simulink model "cllc_control"  (R2022a)
settings: Solver=FixedStepDiscrete  StartTime=0.0  StopTime=Inf  FixedStep=stepsize  RelTol=1e-9  AbsTol=1e-9  EnableMultiTasking=on
model workspace (MAT data in the model file):
  A_d = [1 2 1 2 1 2 1 2 1 2 1 2 ... (18 elements, 2x9)]
  dcdc_direction = 1
  iout_ref : Simulink.Parameter (value not decoded)
  llc1_pri_idc : Simulink.Signal (value not decoded)
  llc1_sec_idc : Simulink.Signal (value not decoded)
  ref_iout : Simulink.Signal (value not decoded)
  ref_iout_calib : Simulink.Signal (value not decoded)
  ref_ss_llc1 : Simulink.Signal (value not decoded)
  ref_vbat : Simulink.Signal (value not decoded)
  ref_vbat_calib : Simulink.Signal (value not decoded)
  vbat : Simulink.Signal (value not decoded)
  vbat_ref : Simulink.Parameter (value not decoded)
  vout : Simulink.Signal (value not decoded)
values from neighbouring files (symbols this model uses):
  epwmclk = 100000000.0    [cllc_data_lib.sldd]
  stepsize = 2.0E-7    [cllc_data_lib.sldd]
  var_dir_v2g = 0.0    [cllc_data_lib.sldd]
undefined symbols (not defined in the file or in its folder): f32Iout, f32VoutTarget
libraries: spsSampleandHoldLib x16, simulink_extras x6
(part 2 of 2)

== system cllc_control/TI_F28379/epwm_cllc1/EPWM_AQCSFRC_SEC_QD ==
  maindrive : Inport
  epwm_aqcsfrc_csf : Inport  Port=2
  synci : Inport  Port=3
  Cast To Boolean : DataTypeConversion  OutDataTypeStr=boolean  SaturateOnIntegerOverflow=off  RndMeth=Floor
  NOT4 : Logic  Operator=NOT  IconShape=distinctive  AllPortsSameDT=off  OutDataTypeStr=boolean
  Product2 : Product
  Sample and Hold1 : spsSampleandHoldLib/Sample and Hold  ic=0  Ts=0
      settings: SourceProductBaseCode=PS
  maindrive' : Outport  PortDimensions=[1 1]
  wires:
  Cast To Boolean/1 -> maindrive'/1
  Sample and Hold1/1 -> Product2/2
  Product2/1 -> Cast To Boolean/1
  synci/1 -> Sample and Hold1/2
  NOT4/1 -> Sample and Hold1/1
  maindrive/1 -> Product2/1
  epwm_aqcsfrc_csf/1 -> NOT4/1

== system cllc_control/TI_F28379/epwm_cllc1/tb_updown ==
  Ts : Inport
  stepsize : Inport  Port=2
  Data Store Memory1 : DataStoreMemory  DataStoreName=sum  ReadBeforeWriteMsg=warning  WriteAfterWriteMsg=warning  WriteAfterReadMsg=warning  ShowAdditionalParam=off  OutDataTypeStr=double
  Data Store Read2 : DataStoreRead  DataStoreName=sum  IndexOptions=Index vector (dialog)  Indices=1  OutputSizes=1
  Data Store Write2 : DataStoreWrite  DataStoreName=sum  IndexOptions=Index vector (dialog)  Indices=1  OutputSizes=1
  MATLAB Function1 : MATLAB Function  Commented=on  TreatAsAtomicUnit=on
  MATLAB Function7 : MATLAB Function  TreatAsAtomicUnit=on
  tb_updown : Outport
  wires:
  Data Store Read2/1 -> MATLAB Function7/1(sum)
  MATLAB Function7/1(updown) -> Data Store Write2/1, tb_updown/1
  Ts/1 -> MATLAB Function7/2(Ts)
  stepsize/1 -> MATLAB Function7/3(stepsize)

== system cllc_control/TI_F28379/epwm_cllc1/tb_updown_ps ==
  Ts : Inport  OutDataTypeStr=double
  stepsize : Inport  Port=2  OutDataTypeStr=double
  synci : Inport  Port=3  OutDataTypeStr=double
  ps : Inport  Port=4  OutDataTypeStr=double
  Data Store Memory1 : DataStoreMemory  DataStoreName=sum2  ReadBeforeWriteMsg=warning  WriteAfterWriteMsg=warning  WriteAfterReadMsg=warning  ShowAdditionalParam=off  OutDataTypeStr=double
  Data Store Read2 : DataStoreRead  DataStoreName=sum2  IndexOptions=Index vector (dialog)  Indices=1  OutputSizes=1
  Data Store Write2 : DataStoreWrite  DataStoreName=sum2  IndexOptions=Index vector (dialog)  Indices=1  OutputSizes=1
  MATLAB Function7 : MATLAB Function  TreatAsAtomicUnit=on
  tb_updown : Outport  OutDataTypeStr=double
  wires:
  stepsize/1 -> MATLAB Function7/3(stepsize)
  Ts/1 -> MATLAB Function7/2(Ts)
  MATLAB Function7/1(updown) -> tb_updown/1, Data Store Write2/1
  Data Store Read2/1 -> MATLAB Function7/1(sum)
  synci/1 -> MATLAB Function7/4(synci)
  ps/1 -> MATLAB Function7/5(ps)

== system cllc_control/TI_F28379/epwm_cllc2/EPWM_AQCSFRC_PRI_QA ==
  maindrive : Inport
  epwm_aqcsfrc_csf : Inport  Port=2
  synci : Inport  Port=3
  Cast To Boolean : DataTypeConversion  OutDataTypeStr=boolean  SaturateOnIntegerOverflow=off  RndMeth=Floor
  NOT4 : Logic  Operator=NOT  IconShape=distinctive  AllPortsSameDT=off  OutDataTypeStr=boolean
  Product2 : Product
  Sample and Hold1 : spsSampleandHoldLib/Sample and Hold  ic=0  Ts=0
      settings: SourceProductBaseCode=PS
  maindrive' : Outport  PortDimensions=[1 1]
  wires:
  Cast To Boolean/1 -> maindrive'/1
  Sample and Hold1/1 -> Product2/2
  Product2/1 -> Cast To Boolean/1
  synci/1 -> Sample and Hold1/2
  NOT4/1 -> Sample and Hold1/1
  maindrive/1 -> Product2/1
  epwm_aqcsfrc_csf/1 -> NOT4/1

== system cllc_control/TI_F28379/epwm_cllc2/EPWM_AQCSFRC_PRI_QB ==
  maindrive : Inport
  epwm_aqcsfrc_csf : Inport  Port=2
  synci : Inport  Port=3
  Cast To Boolean : DataTypeConversion  OutDataTypeStr=boolean  SaturateOnIntegerOverflow=off  RndMeth=Floor
  NOT4 : Logic  Operator=NOT  IconShape=distinctive  AllPortsSameDT=off  OutDataTypeStr=boolean
  Product2 : Product
  Sample and Hold1 : spsSampleandHoldLib/Sample and Hold  ic=0  Ts=0
      settings: SourceProductBaseCode=PS
  maindrive' : Outport  PortDimensions=[1 1]
  wires:
  Cast To Boolean/1 -> maindrive'/1
  epwm_aqcsfrc_csf/1 -> NOT4/1
  maindrive/1 -> Product2/1
  NOT4/1 -> Sample and Hold1/1
  synci/1 -> Sample and Hold1/2
  Product2/1 -> Cast To Boolean/1
  Sample and Hold1/1 -> Product2/2

== system cllc_control/TI_F28379/epwm_cllc2/EPWM_AQCSFRC_PRI_QC ==
  maindrive : Inport
  epwm_aqcsfrc_csf : Inport  Port=2
  synci : Inport  Port=3
  Cast To Boolean : DataTypeConversion  OutDataTypeStr=boolean  SaturateOnIntegerOverflow=off  RndMeth=Floor
  NOT4 : Logic  Operator=NOT  IconShape=distinctive  AllPortsSameDT=off  OutDataTypeStr=boolean
  Product2 : Product
  Sample and Hold1 : spsSampleandHoldLib/Sample and Hold  ic=0  Ts=0
      settings: SourceProductBaseCode=PS
  maindrive' : Outport  PortDimensions=[1 1]
  wires:
  Cast To Boolean/1 -> maindrive'/1
  epwm_aqcsfrc_csf/1 -> NOT4/1
  maindrive/1 -> Product2/1
  NOT4/1 -> Sample and Hold1/1
  synci/1 -> Sample and Hold1/2
  Product2/1 -> Cast To Boolean/1
  Sample and Hold1/1 -> Product2/2

== system cllc_control/TI_F28379/epwm_cllc2/EPWM_AQCSFRC_PRI_QD ==
  maindrive : Inport
  epwm_aqcsfrc_csf : Inport  Port=2
  synci : Inport  Port=3
  Cast To Boolean : DataTypeConversion  OutDataTypeStr=boolean  SaturateOnIntegerOverflow=off  RndMeth=Floor
  NOT4 : Logic  Operator=NOT  IconShape=distinctive  AllPortsSameDT=off  OutDataTypeStr=boolean
  Product2 : Product
  Sample and Hold1 : spsSampleandHoldLib/Sample and Hold  ic=0  Ts=0
      settings: SourceProductBaseCode=PS
  maindrive' : Outport  PortDimensions=[1 1]
  wires:
  Cast To Boolean/1 -> maindrive'/1
  Sample and Hold1/1 -> Product2/2
  Product2/1 -> Cast To Boolean/1
  synci/1 -> Sample and Hold1/2
  NOT4/1 -> Sample and Hold1/1
  maindrive/1 -> Product2/1
  epwm_aqcsfrc_csf/1 -> NOT4/1

== system cllc_control/TI_F28379/epwm_cllc2/EPWM_AQCSFRC_SEC_QA ==
  maindrive : Inport
  epwm_aqcsfrc_csf : Inport  Port=2
  synci : Inport  Port=3
  Cast To Boolean : DataTypeConversion  OutDataTypeStr=boolean  SaturateOnIntegerOverflow=off  RndMeth=Floor
  NOT4 : Logic  Operator=NOT  IconShape=distinctive  AllPortsSameDT=off  OutDataTypeStr=boolean
  Product2 : Product
  Sample and Hold1 : spsSampleandHoldLib/Sample and Hold  ic=0  Ts=0
      settings: SourceProductBaseCode=PS
  maindrive' : Outport  PortDimensions=[1 1]
  wires:
  epwm_aqcsfrc_csf/1 -> NOT4/1
  maindrive/1 -> Product2/1
  NOT4/1 -> Sample and Hold1/1
  synci/1 -> Sample and Hold1/2
  Product2/1 -> Cast To Boolean/1
  Sample and Hold1/1 -> Product2/2
  Cast To Boolean/1 -> maindrive'/1

== system cllc_control/TI_F28379/epwm_cllc2/EPWM_AQCSFRC_SEC_QB ==
  maindrive : Inport
  epwm_aqcsfrc_csf : Inport  Port=2
  synci : Inport  Port=3
  Cast To Boolean : DataTypeConversion  OutDataTypeStr=boolean  SaturateOnIntegerOverflow=off  RndMeth=Floor
  NOT4 : Logic  Operator=NOT  IconShape=distinctive  AllPortsSameDT=off  OutDataTypeStr=boolean
  Product2 : Product
  Sample and Hold1 : spsSampleandHoldLib/Sample and Hold  ic=0  Ts=0
      settings: SourceProductBaseCode=PS
  maindrive' : Outport  PortDimensions=[1 1]
  wires:
  Sample and Hold1/1 -> Product2/2
  Product2/1 -> Cast To Boolean/1
  synci/1 -> Sample and Hold1/2
  NOT4/1 -> Sample and Hold1/1
  maindrive/1 -> Product2/1
  epwm_aqcsfrc_csf/1 -> NOT4/1
  Cast To Boolean/1 -> maindrive'/1

== system cllc_control/TI_F28379/epwm_cllc2/EPWM_AQCSFRC_SEC_QC ==
  maindrive : Inport
  epwm_aqcsfrc_csf : Inport  Port=2
  synci : Inport  Port=3
  Cast To Boolean : DataTypeConversion  OutDataTypeStr=boolean  SaturateOnIntegerOverflow=off  RndMeth=Floor
  NOT4 : Logic  Operator=NOT  IconShape=distinctive  AllPortsSameDT=off  OutDataTypeStr=boolean
  Product2 : Product
  Sample and Hold1 : spsSampleandHoldLib/Sample and Hold  ic=0  Ts=0
      settings: SourceProductBaseCode=PS
  maindrive' : Outport  PortDimensions=[1 1]
  wires:
  Sample and Hold1/1 -> Product2/2
  Product2/1 -> Cast To Boolean/1
  synci/1 -> Sample and Hold1/2
  NOT4/1 -> Sample and Hold1/1
  maindrive/1 -> Product2/1
  epwm_aqcsfrc_csf/1 -> NOT4/1
  Cast To Boolean/1 -> maindrive'/1

== system cllc_control/TI_F28379/epwm_cllc2/EPWM_AQCSFRC_SEC_QD ==
  maindrive : Inport
  epwm_aqcsfrc_csf : Inport  Port=2
  synci : Inport  Port=3
  Cast To Boolean : DataTypeConversion  OutDataTypeStr=boolean  SaturateOnIntegerOverflow=off  RndMeth=Floor
  NOT4 : Logic  Operator=NOT  IconShape=distinctive  AllPortsSameDT=off  OutDataTypeStr=boolean
  Product2 : Product
  Sample and Hold1 : spsSampleandHoldLib/Sample and Hold  ic=0  Ts=0
      settings: SourceProductBaseCode=PS
  maindrive' : Outport  PortDimensions=[1 1]
  wires:
  epwm_aqcsfrc_csf/1 -> NOT4/1
  maindrive/1 -> Product2/1
  NOT4/1 -> Sample and Hold1/1
  synci/1 -> Sample and Hold1/2
  Product2/1 -> Cast To Boolean/1
  Sample and Hold1/1 -> Product2/2
  Cast To Boolean/1 -> maindrive'/1

== system cllc_control/TI_F28379/epwm_cllc2/tb_updown ==
  Ts : Inport
  stepsize : Inport  Port=2
  Data Store Memory1 : DataStoreMemory  DataStoreName=sum  ReadBeforeWriteMsg=warning  WriteAfterWriteMsg=warning  WriteAfterReadMsg=warning  ShowAdditionalParam=off  OutDataTypeStr=double
  Data Store Read2 : DataStoreRead  DataStoreName=sum  IndexOptions=Index vector (dialog)  Indices=1  OutputSizes=1
  Data Store Write2 : DataStoreWrite  DataStoreName=sum  IndexOptions=Index vector (dialog)  Indices=1  OutputSizes=1
  MATLAB Function1 : MATLAB Function  Commented=on  TreatAsAtomicUnit=on
  MATLAB Function7 : MATLAB Function  TreatAsAtomicUnit=on
  tb_updown : Outport
  wires:
  stepsize/1 -> MATLAB Function7/3(stepsize)
  Ts/1 -> MATLAB Function7/2(Ts)
  MATLAB Function7/1(updown) -> tb_updown/1, Data Store Write2/1
  Data Store Read2/1 -> MATLAB Function7/1(sum)

== system cllc_control/TI_F28379/epwm_cllc2/tb_updown_ps ==
  Ts : Inport
  stepsize : Inport  Port=2
  synci : Inport  Port=3
  ps : Inport  Port=4
  Data Store Memory1 : DataStoreMemory  DataStoreName=sum2  ReadBeforeWriteMsg=warning  WriteAfterWriteMsg=warning  WriteAfterReadMsg=warning  ShowAdditionalParam=off  OutDataTypeStr=double
  Data Store Read2 : DataStoreRead  DataStoreName=sum2  IndexOptions=Index vector (dialog)  Indices=1  OutputSizes=1
  Data Store Write2 : DataStoreWrite  DataStoreName=sum2  IndexOptions=Index vector (dialog)  Indices=1  OutputSizes=1
  MATLAB Function7 : MATLAB Function  TreatAsAtomicUnit=on
  tb_updown : Outport
  wires:
  ps/1 -> MATLAB Function7/5(ps)
  synci/1 -> MATLAB Function7/4(synci)
  Data Store Read2/1 -> MATLAB Function7/1(sum)
  MATLAB Function7/1(updown) -> Data Store Write2/1, tb_updown/1
  Ts/1 -> MATLAB Function7/2(Ts)
  stepsize/1 -> MATLAB Function7/3(stepsize)

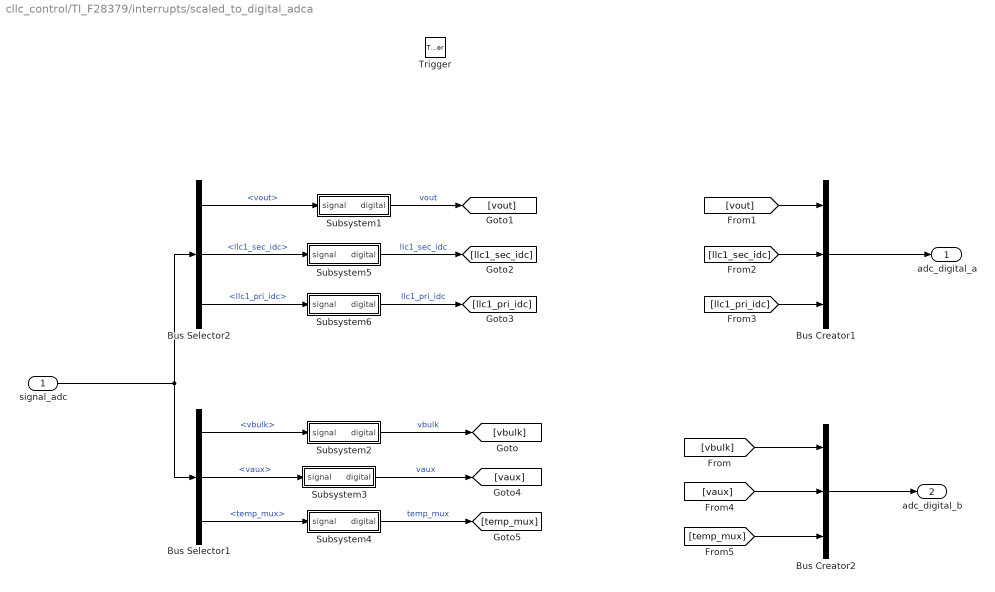
== system cllc_control/TI_F28379/interrupts/scaled_to_digital_adca ==
  signal_adc : Inport
  Trigger : TriggerPort  VariantControl=Variant  PortDimensions=1
  Bus Creator1 : BusCreator  Inputs=3  OutDataTypeStr=Bus: adca_digital  NonVirtualBus=on
  Bus Creator2 : BusCreator  Inputs=3  OutDataTypeStr=Bus: adcb_digital  NonVirtualBus=on
  Bus Selector1 : BusSelector  OutputSignals=vbulk,vaux,temp_mux
  Bus Selector2 : BusSelector  OutputSignals=vout,llc1_sec_idc,llc1_pri_idc
  Subsystem1 : Subsystem
  Subsystem2 : Subsystem
  Subsystem3 : Subsystem
  Subsystem4 : Subsystem
  Subsystem5 : Subsystem
  Subsystem6 : Subsystem
  adc_digital_a : Outport
  adc_digital_b : Outport  Port=2
  wires:
  Bus Creator1/1 -> adc_digital_a/1
  Bus Selector2/1 -> Subsystem1/1(signal)  "<vout>"
  Bus Selector2/2 -> Subsystem5/1(signal)  "<llc1_sec_idc>"
  Bus Selector2/3 -> Subsystem6/1(signal)  "<llc1_pri_idc>"
  Subsystem1/1(digital) -> [vout]  "vout"
  Subsystem5/1(digital) -> [llc1_sec_idc]  "llc1_sec_idc"
  Subsystem6/1(digital) -> [llc1_pri_idc]  "llc1_pri_idc"
  [llc1_pri_idc] -> Bus Creator1/3
  [llc1_sec_idc] -> Bus Creator1/2
  [vout] -> Bus Creator1/1
  [vaux] -> Bus Creator2/2
  Bus Selector1/2 -> Subsystem3/1(signal)  "<vaux>"
  Bus Creator2/1 -> adc_digital_b/1
  [temp_mux] -> Bus Creator2/3
  Bus Selector1/3 -> Subsystem4/1(signal)  "<temp_mux>"
  [vbulk] -> Bus Creator2/1
  signal_adc/1 -> Bus Selector2/1, Bus Selector1/1
  Subsystem2/1(digital) -> [vbulk]  "vbulk"
  Subsystem4/1(digital) -> [temp_mux]  "temp_mux"
  Subsystem3/1(digital) -> [vaux]  "vaux"
  Bus Selector1/1 -> Subsystem2/1(signal)  "<vbulk>"

== system cllc_control/TI_F28379/interrupts/scaled_to_digital_adca/Subsystem1 ==
  note: Sampling
  note: ADC
      | Quantization
  signal : Inport
  Idealized ADC quantizer1 : simulink_extras/Additional Discrete/Idealized ADC quantizer  NumberOfConverterBits=12  Vmin=0  Vmax=3.3  OutputDataType=uint16  OutputNegativeValues=off
  Zero-Order Hold1 : ZeroOrderHold  SampleTime=-1
  digital : Outport
  wires:
  signal/1 -> Zero-Order Hold1/1
  Idealized ADC quantizer1/1 -> digital/1
  Zero-Order Hold1/1 -> Idealized ADC quantizer1/1

== system cllc_control/TI_F28379/interrupts/scaled_to_digital_adca/Subsystem2 ==
  note: Sampling
  note: ADC
      | Quantization
  signal : Inport
  Idealized ADC quantizer1 : simulink_extras/Additional Discrete/Idealized ADC quantizer  NumberOfConverterBits=12  Vmin=0  Vmax=3.3  OutputDataType=uint16  OutputNegativeValues=off
  Zero-Order Hold1 : ZeroOrderHold  SampleTime=-1
  digital : Outport
  wires:
  signal/1 -> Zero-Order Hold1/1
  Idealized ADC quantizer1/1 -> digital/1
  Zero-Order Hold1/1 -> Idealized ADC quantizer1/1

== system cllc_control/TI_F28379/interrupts/scaled_to_digital_adca/Subsystem3 ==
  note: ADC
      | Quantization
  note: Sampling
  signal : Inport
  Idealized ADC quantizer1 : simulink_extras/Additional Discrete/Idealized ADC quantizer  NumberOfConverterBits=12  Vmin=0  Vmax=3.3  OutputDataType=uint16  OutputNegativeValues=off
  Zero-Order Hold1 : ZeroOrderHold  SampleTime=-1
  digital : Outport
  wires:
  Zero-Order Hold1/1 -> Idealized ADC quantizer1/1
  Idealized ADC quantizer1/1 -> digital/1
  signal/1 -> Zero-Order Hold1/1

== system cllc_control/TI_F28379/interrupts/scaled_to_digital_adca/Subsystem4 ==
  note: Sampling
  note: ADC
      | Quantization
  signal : Inport
  Idealized ADC quantizer1 : simulink_extras/Additional Discrete/Idealized ADC quantizer  NumberOfConverterBits=12  Vmin=0  Vmax=3.3  OutputDataType=uint16  OutputNegativeValues=off
  Zero-Order Hold1 : ZeroOrderHold  SampleTime=-1
  digital : Outport
  wires:
  signal/1 -> Zero-Order Hold1/1
  Idealized ADC quantizer1/1 -> digital/1
  Zero-Order Hold1/1 -> Idealized ADC quantizer1/1

== system cllc_control/TI_F28379/interrupts/scaled_to_digital_adca/Subsystem5 ==
  note: Sampling
  note: ADC
      | Quantization
  signal : Inport
  Idealized ADC quantizer1 : simulink_extras/Additional Discrete/Idealized ADC quantizer  NumberOfConverterBits=12  Vmin=0  Vmax=3.3  OutputDataType=uint16  OutputNegativeValues=off
  Zero-Order Hold1 : ZeroOrderHold  SampleTime=-1
  digital : Outport
  wires:
  signal/1 -> Zero-Order Hold1/1
  Idealized ADC quantizer1/1 -> digital/1
  Zero-Order Hold1/1 -> Idealized ADC quantizer1/1

== system cllc_control/TI_F28379/interrupts/scaled_to_digital_adca/Subsystem6 ==
  note: ADC
      | Quantization
  note: Sampling
  signal : Inport
  Idealized ADC quantizer1 : simulink_extras/Additional Discrete/Idealized ADC quantizer  NumberOfConverterBits=12  Vmin=0  Vmax=3.3  OutputDataType=uint16  OutputNegativeValues=off
  Zero-Order Hold1 : ZeroOrderHold  SampleTime=-1
  digital : Outport
  wires:
  Zero-Order Hold1/1 -> Idealized ADC quantizer1/1
  Idealized ADC quantizer1/1 -> digital/1
  signal/1 -> Zero-Order Hold1/1

== matlab function cllc_control/TI_F28379/epwm_cllc2/epwm1 ==
  data: PWMA output; timebase input; Ts input; CMPA input; CMPB input; PWMB output; deadband input; stepsize input; epwmclk input; SYNCOUT output
function [PWMA, PWMB, SYNCOUT] = fcn(timebase, Ts, CMPA, CMPB, deadband, stepsize, epwmclk)

persistent count_up;
if(isempty(count_up))
    count_up=1;
end

if(timebase > (Ts-stepsize))
    count_up=-1;
elseif(timebase < abs(stepsize))
    count_up=1;
end

CMPA=CMPA/epwmclk;
CMPB=CMPB/epwmclk;
deadband=deadband/epwmclk;

if(count_up==1)
    if(timebase>=single(0) && timebase<single(CMPB-deadband))
        PWMA=1;
        PWMB=0;
    else
        PWMA=0;
        PWMB=0;
    end
elseif(count_up==-1)
    if(timebase<=(Ts) && timebase>single(CMPA+deadband))
        PWMA=0;
        PWMB=1;
    else
        PWMA=0;
        PWMB=0;
    end
else
    PWMA=0;
    PWMB=0;
end

if(timebase>=single(0) && timebase<stepsize)
    SYNCOUT=1;
else
    SYNCOUT=0;
end
    
end

== matlab function cllc_control/TI_F28379/epwm_cllc1/center-aligned_high_freq_sw1 ==
  data: PWMA output; timebase input; Ts input; CMPA input; CMPB input; PWMB output; deadband input; stepsize input; epwmclk input; SYNCOUT output
function [PWMA, PWMB, SYNCOUT] = fcn(timebase, Ts, CMPA,CMPB, deadband, stepsize, epwmclk)

persistent CMPAU;
persistent CMPAD; 
persistent CMPBU;
persistent CMPBD;
persistent margin;

persistent count_up;
if(isempty(count_up))
    count_up=1;
end

if(timebase > (Ts-stepsize))
    count_up=-1;
elseif(timebase < abs(stepsize))
    count_up=1;
end

%Step 1. Convert input parameters to time domain
deadband = deadband/epwmclk;
margin = single(1/epwmclk);

%Step 2. Calculate CMPAU, CMPBU, CMPBD, CMPAD in time domain
CMPAU = Ts/2 - deadband/2;
CMPBU = Ts/2 + deadband/2;
CMPBD = Ts + CMPAU;
CMPAD = Ts + CMPBU;

%Step 3. Output PWM
%At 0<=timebase<Ts
if(timebase >= single(0) && timebase < single(CMPAU-margin))
    PWMA=0;
    PWMB=1;
elseif(timebase >= CMPBU && timebase < single(Ts-margin))
    PWMA=1;
    PWMB=0;
%At Ts<=timebase<2Ts
elseif(timebase >= Ts && timebase < single(CMPBD-margin))
    PWMA=1;
    PWMB=0;       
elseif(timebase >= CMPAD && timebase < single(2*Ts-margin))
    PWMA=0;
    PWMB=1;
%At deadtime
else 
    PWMA=0; 
    PWMB=0; 
end

%Step 4. Assert SYNCOUT at tbctr = zero 
if(timebase>=single(0) && timebase<stepsize)
    SYNCOUT=1;
else
    SYNCOUT=0;
end
    
end

== matlab function cllc_control/TI_F28379/epwm_cllc1/tb_updown/MATLAB Function1 ==
  data: updown output; sum input; Ts input; stepsize input
function updown = fcn(sum, Ts, stepsize)

persistent signed_stepsize;
if(isempty(signed_stepsize))
    signed_stepsize = stepsize;
end

sum = sum + signed_stepsize;

if(sum > (Ts-signed_stepsize) || sum < abs(signed_stepsize))
    signed_stepsize = -1*signed_stepsize;
end

updown = sum;

== matlab function cllc_control/TI_F28379/epwm_cllc2/tb_updown/MATLAB Function1 ==
  data: updown output; sum input; Ts input; stepsize input
function updown = fcn(sum, Ts, stepsize)

persistent signed_stepsize;
if(isempty(signed_stepsize))
    signed_stepsize = stepsize;
end

sum = sum + signed_stepsize;

if(sum > (Ts-signed_stepsize) || sum < abs(signed_stepsize))
    signed_stepsize = -1*signed_stepsize;
end

updown = sum;

== stateflow chart cllc_control/TI_F28379/clb1/sr_control ==
  state STAGE1_2 [parallel]
    settings: executionOrder=1
    note: Digital filter for SR ON
    note: Utilize 2 comparators for custom hysteresis
    state INIT
      en:
      cmp_sr_filt = 0;
    state VALID_ON_CMPH
      en:
      cmp_sr_filt = 1;
    (default) -> STAGE1_2.INIT
    VALID_ON_CMPH -> STAGE1_2.INIT : [cmp_sr<5]
    STAGE1_2.INIT -> VALID_ON_CMPH : [duration((cmp_sr>8) > 120e-9)]
  state STAGE3 [parallel]
    settings: executionOrder=2
    note: Limit one SR pulse per one cycle of main drive PWM
    state INIT
      en:
      pwm_sr = 0;
    state EN_SR
      en:
      pwm_sr = 1;
    state DIS_SR
      en:
      pwm_sr = 0;
    (default) -> STAGE3.INIT
    DIS_SR -> STAGE3.INIT : [pwm_md]
    STAGE3.INIT -> EN_SR : [cmp_sr_filt == 1]
    EN_SR -> DIS_SR : [cmp_sr_filt == 0]
  data: cmp_sr input single; pwm_md input; pwm_sr output; cmp_sr_filt local uint8 size=[1]

== stateflow chart cllc_control/TI_F28379/clb2/sr_control ==
  state STAGE1_2 [parallel]
    settings: executionOrder=1
    note: Digital filter for SR ON
    note: Utilize 2 comparators for custom hysteresis
    state INIT
      en:
      cmp_sr_filt = 0;
    state VALID_ON_CMPH
      en:
      cmp_sr_filt = 1;
    (default) -> STAGE1_2.INIT
    VALID_ON_CMPH -> STAGE1_2.INIT : [cmp_sr>-5]
    STAGE1_2.INIT -> VALID_ON_CMPH : [duration((cmp_sr<-8) > 120e-9)]
  state STAGE3 [parallel]
    settings: executionOrder=2
    note: Limit one SR pulse per one cycle of main drive PWM
    state INIT
      en:
      pwm_sr = 0;
    state EN_SR
      en:
      pwm_sr = 1;
    state DIS_SR
      en:
      pwm_sr = 0;
    (default) -> STAGE3.INIT
    DIS_SR -> STAGE3.INIT : [pwm_md]
    STAGE3.INIT -> EN_SR : [cmp_sr_filt == 1]
    EN_SR -> DIS_SR : [cmp_sr_filt == 0]
  data: cmp_sr input single; pwm_md input; pwm_sr output; cmp_sr_filt local uint8 size=[1]

== stateflow chart cllc_control/TI_F28379/clb1/pwm_md_trig/Chart ==
  state INIT
    en:
    OUT=1;
  state ST2
    en:
    OUT=0;
  (default) -> INIT
  INIT -> ST2
  data: OUT output boolean

== stateflow chart cllc_control/TI_F28379/clb2/pwm_md_trig/Chart ==
  state INIT
    en:
    OUT=1;
  state ST2
    en:
    OUT=0;
  (default) -> INIT
  INIT -> ST2
  data: OUT output boolean

== matlab function cllc_control/TI_F28379/epwm_cllc2/tb_updown/MATLAB Function7 ==
  data: updown output; sum input; Ts input; stepsize input
function updown = fcn(sum, Ts, stepsize)

persistent signed_stepsize;
if(isempty(signed_stepsize))
    signed_stepsize = stepsize;
end

sum = sum + signed_stepsize;

if(sum > (Ts-signed_stepsize))
    signed_stepsize = -1*stepsize;
elseif(sum < abs(signed_stepsize))
    signed_stepsize = stepsize;
end

updown = sum;

== matlab function cllc_control/TI_F28379/epwm_cllc2/tb_updown_ps/MATLAB Function7 ==
  data: updown output; sum input; Ts input; stepsize input; synci input; ps input
function updown = fcn(sum, Ts, stepsize, synci, ps)

persistent signed_stepsize;
if(isempty(signed_stepsize))
    signed_stepsize = stepsize;
end

sum = sum + signed_stepsize;

if(~synci)
    if(sum > (Ts-signed_stepsize))
        signed_stepsize = -1*stepsize;
    elseif(sum < abs(signed_stepsize))
        signed_stepsize = stepsize;
    end
else
    if(ps~=0)
        sum=ps;
        signed_stepsize = -1*stepsize;
    else
        sum=ps;
        signed_stepsize = stepsize;
    end
end

updown = sum;

== stateflow chart cllc_control/TI_F28379/interrupts/Chart2 ==
  state INT_ADCA [parallel]
    settings: executionOrder=1
    state INIT
    state FUNCTION_CALL
      en:
      int_adca;
      int_adcb;
    (default) -> INT_ADCA.INIT
    INT_ADCA.FUNCTION_CALL -> INT_ADCA.INIT : [!tbctr_cllc1]
    INT_ADCA.INIT -> INT_ADCA.FUNCTION_CALL : [tbctr_cllc1]
  state INT_CANRX [parallel]
    settings: executionOrder=2
    state INIT
      en:
      cnt_50us=1;
    state FUNCTION_CALL
      en:
      int_canrx;
    (default) -> INT_CANRX.INIT
    INT_CANRX.FUNCTION_CALL -> INT_CANRX.INIT : {cnt_50us=0;}
    INT_CANRX.INIT -> INT_CANRX.FUNCTION_CALL : [duration(cnt_50us>0)>50e-6]
  data: tbctr_cllc1 input single; cnt_50us local uint8 =0
  events: int_adca output FUNCTION_CALL_EVENT; int_adcb output FUNCTION_CALL_EVENT; int_canrx output FUNCTION_CALL_EVENT

== matlab function cllc_control/TI_F28379/epwm_cllc1/epwm ==
  data: PWMA output; timebase input; Ts input; CMPA input; CMPB input; PWMB output; deadband input; stepsize input; epwmclk input; SYNCOUT output
function [PWMA, PWMB, SYNCOUT] = fcn(timebase, Ts, CMPA, CMPB, deadband, stepsize, epwmclk)

persistent count_up;
if(isempty(count_up))
    count_up=1;
end

if(timebase > (Ts-stepsize))
    count_up=-1;
elseif(timebase < abs(stepsize))
    count_up=1;
end

CMPA=CMPA/epwmclk;
CMPB=CMPB/epwmclk;
deadband=deadband/epwmclk;
margin = 1/epwmclk;

if(count_up==1)
    if(timebase>=single(0) && timebase<single(CMPB-deadband+margin))
        PWMA=1;
        PWMB=0;
    else
        PWMA=0;
        PWMB=0;
    end
elseif(count_up==-1)
    if(timebase<=(Ts) && timebase>single(CMPA+deadband-margin))
        PWMA=0;
        PWMB=1;
    else
        PWMA=0;
        PWMB=0;
    end
else
    PWMA=0;
    PWMB=0;
end

if(timebase>=single(0) && timebase<stepsize)
    SYNCOUT=1;
else
    SYNCOUT=0;
end
    
end

== stateflow chart cllc_control/TI_F28379/50us ==
  state INIT
    en:
    sim_control;
  (default) -> INIT
  INIT -> INIT
  events: sim_control output FUNCTION_CALL_EVENT

== matlab function cllc_control/TI_F28379/epwm_cllc1/epwm1 ==
  data: PWMA output; timebase input; Ts input; CMPA input; CMPB input; PWMB output; deadband input; stepsize input; epwmclk input; SYNCOUT output
function [PWMA, PWMB, SYNCOUT] = fcn(timebase, Ts, CMPA, CMPB, deadband, stepsize, epwmclk)

persistent count_up;
if(isempty(count_up))
    count_up=1;
end

if(timebase > (Ts-stepsize))
    count_up=-1;
elseif(timebase < abs(stepsize))
    count_up=1;
end

CMPA=CMPA/epwmclk;
CMPB=CMPB/epwmclk;
deadband=deadband/epwmclk;
margin = 1/epwmclk;

if(count_up==1)
    if(timebase>=single(0) && timebase<single(CMPB-deadband + margin))
        PWMA=1;
        PWMB=0;
    else
        PWMA=0;
        PWMB=0;
    end
elseif(count_up==-1)
    if(timebase<=(Ts) && timebase>single(CMPA+deadband - margin))
        PWMA=0;
        PWMB=1;
    else
        PWMA=0;
        PWMB=0;
    end
else
    PWMA=0;
    PWMB=0;
end

if(timebase>=single(0) && timebase<stepsize)
    SYNCOUT=1;
else
    SYNCOUT=0;
end
    
end

== matlab function cllc_control/TI_F28379/epwm_cllc1/tb_updown/MATLAB Function7 ==
  data: updown output; sum input; Ts input; stepsize input
function updown = fcn(sum, Ts, stepsize)

persistent signed_stepsize;
if(isempty(signed_stepsize))
    signed_stepsize = stepsize;
end

sum = sum + signed_stepsize;

if(sum > (Ts-signed_stepsize))
    signed_stepsize = -1*stepsize;
elseif(sum <= abs(signed_stepsize))
    signed_stepsize = stepsize;
end

updown = sum;

== matlab function cllc_control/TI_F28379/epwm_cllc1/tb_updown_ps/MATLAB Function7 ==
  data: updown output; sum input; Ts input; stepsize input; synci input; ps input
function updown = fcn(sum, Ts, stepsize, synci, ps)

persistent signed_stepsize;
if(isempty(signed_stepsize))
    signed_stepsize = stepsize;
end

sum = sum + signed_stepsize;

if(~synci)
    if(sum > (Ts-signed_stepsize))
        signed_stepsize = -1*stepsize;
    elseif(sum <= 0)%abs(signed_stepsize))
        signed_stepsize = stepsize;
    end
else
    if(ps~=0)
        sum=ps;
        signed_stepsize = -1*stepsize;
    else
        sum=ps;
        signed_stepsize = stepsize;
    end
end

updown = sum;

if(updown <= 0)
    updown =0;
end

== stateflow chart cllc_control/TI_F28379/clb3/sr_control ==
  state STAGE1_2 [parallel]
    settings: executionOrder=1
    note: Digital filter for SR ON
    note: Utilize 2 comparators for custom hysteresis
    state INIT
      en:
      cmp_sr_filt = 0;
    state VALID_ON_CMPH
      en:
      cmp_sr_filt = 1;
    (default) -> STAGE1_2.INIT
    VALID_ON_CMPH -> STAGE1_2.INIT : [cmp_sr<5]
    STAGE1_2.INIT -> VALID_ON_CMPH : [duration((cmp_sr>8) > 120e-9)]
  state STAGE3 [parallel]
    settings: executionOrder=2
    note: Limit one SR pulse per one cycle of main drive PWM
    state INIT
      en:
      pwm_sr = 0;
    state EN_SR
      en:
      pwm_sr = 1;
    state DIS_SR
      en:
      pwm_sr = 0;
    (default) -> STAGE3.INIT
    DIS_SR -> STAGE3.INIT : [pwm_md]
    STAGE3.INIT -> EN_SR : [cmp_sr_filt == 1]
    EN_SR -> DIS_SR : [cmp_sr_filt == 0]
  data: cmp_sr input single; pwm_md input; pwm_sr output; cmp_sr_filt local uint8 size=[1]

== stateflow chart cllc_control/TI_F28379/clb3/pwm_md_trig/Chart ==
  state INIT
    en:
    OUT=1;
  state ST2
    en:
    OUT=0;
  (default) -> INIT
  INIT -> ST2
  data: OUT output boolean

== stateflow chart cllc_control/TI_F28379/clb4/sr_control ==
  state STAGE1_2 [parallel]
    settings: executionOrder=1
    note: Digital filter for SR ON
    note: Utilize 2 comparators for custom hysteresis
    state INIT
      en:
      cmp_sr_filt = 0;
    state VALID_ON_CMPH
      en:
      cmp_sr_filt = 1;
    (default) -> STAGE1_2.INIT
    VALID_ON_CMPH -> STAGE1_2.INIT : [cmp_sr>-5]
    STAGE1_2.INIT -> VALID_ON_CMPH : [duration((cmp_sr<-8) > 120e-9)]
  state STAGE3 [parallel]
    settings: executionOrder=2
    note: Limit one SR pulse per one cycle of main drive PWM
    state INIT
      en:
      pwm_sr = 0;
    state EN_SR
      en:
      pwm_sr = 1;
    state DIS_SR
      en:
      pwm_sr = 0;
    (default) -> STAGE3.INIT
    DIS_SR -> STAGE3.INIT : [pwm_md]
    STAGE3.INIT -> EN_SR : [cmp_sr_filt == 1]
    EN_SR -> DIS_SR : [cmp_sr_filt == 0]
  data: cmp_sr input single; pwm_md input; pwm_sr output; cmp_sr_filt local uint8 size=[1]

== stateflow chart cllc_control/TI_F28379/clb4/pwm_md_trig/Chart ==
  state INIT
    en:
    OUT=1;
  state ST2
    en:
    OUT=0;
  (default) -> INIT
  INIT -> ST2
  data: OUT output boolean

== stateflow chart cllc_control/TI_F28379/100us ==
  state INIT
    en:
    sim_idletask;
  (default) -> INIT
  INIT -> INIT
  events: sim_idletask output FUNCTION_CALL_EVENT

== matlab function cllc_control/TI_F28379/epwm_cllc1/center-aligned_high_freq_sw2 ==
  data: PWMA output; timebase input; Ts input; CMPA input; CMPB input; PWMB output; deadband input; stepsize input; epwmclk input; SYNCOUT output
function [PWMA, PWMB, SYNCOUT] = fcn(timebase, Ts, CMPA,CMPB, deadband, stepsize, epwmclk)

persistent CMPAU;
persistent CMPAD; 
persistent CMPBU;
persistent CMPBD;
persistent margin;

%Step 1. Convert input parameters to time domain
deadband = deadband/epwmclk;
margin = single(1/epwmclk);

%Step 2. Calculate CMPAU, CMPBU, CMPBD, CMPAD in time domain
CMPAU = Ts/2 - deadband/2;
CMPBU = Ts/2 + deadband/2;
CMPBD = Ts + CMPAU;
CMPAD = Ts + CMPBU;

%Step 3. Output PWM
%At 0<=timebase<Ts
if(timebase >= single(0) && timebase < single(CMPAU-margin))
    PWMA=0;
    PWMB=1;
elseif(timebase >= CMPBU && timebase < single(Ts-margin))
    PWMA=1;
    PWMB=0;
%At Ts<=timebase<2Ts
elseif(timebase >= Ts && timebase < single(CMPBD-margin))
    PWMA=1;
    PWMB=0;       
elseif(timebase >= CMPAD && timebase < single(2*Ts-margin))
    PWMA=0;
    PWMB=1;
%At deadtime
else 
    PWMA=0; 
    PWMB=0; 
end

%Step 4. Assert SYNCOUT at tbctr = zero 
if(timebase>=single(0) && timebase<stepsize)
    SYNCOUT=1;
else
    SYNCOUT=0;
end
    
end

== matlab function cllc_control/TI_F28379/epwm_cllc2/epwm ==
  data: PWMA output; timebase input; Ts input; CMPA input; CMPB input; PWMB output; deadband input; stepsize input; epwmclk input; SYNCOUT output
function [PWMA, PWMB, SYNCOUT] = fcn(timebase, Ts, CMPA, CMPB, deadband, stepsize, epwmclk)

persistent count_up;
if(isempty(count_up))
    count_up=1;
end

if(timebase > (Ts-stepsize))
    count_up=-1;
elseif(timebase < abs(stepsize))
    count_up=1;
end

CMPA=CMPA/epwmclk;
CMPB=CMPB/epwmclk;
deadband=deadband/epwmclk;

if(count_up==1)
    if(timebase>=single(0) && timebase<single(CMPB-deadband))
        PWMA=1;
        PWMB=0;
    else
        PWMA=0;
        PWMB=0;
    end
elseif(count_up==-1)
    if(timebase<=(Ts) && timebase>single(CMPA+deadband))
        PWMA=0;
        PWMB=1;
    else
        PWMA=0;
        PWMB=0;
    end
else
    PWMA=0;
    PWMB=0;
end

if(timebase>=single(0) && timebase<stepsize)
    SYNCOUT=1;
else
    SYNCOUT=0;
end
    
end
